simulink model "Model_sim"  (R2018b)
settings: Solver=ode3  StartTime=0.0  StopTime=0.08  FixedStep=0.02  RelTol=1e-3
values from neighbouring files (symbols this model uses):
  q1_d_in = xd0(1,2)    [Project.m]    (also in definitivo.mat = -0.537500213816)
  q1_in = xi0(1,2)    [Project.m]    (also in definitivo.mat = 4.84978546313)
  q2_d_in = xd0(2,2)    [Project.m]    (also in definitivo.mat = 1.25712801049)
  q2_in = xi0(2,2)    [Project.m]    (also in definitivo.mat = 0.122900974203)
  Ts = 1/fs    (= 0.02)    [Project.m]    (also in definitivo.mat)
settings Model: Creator=Andrea Ghezzi  LastModifiedBy=sl65b

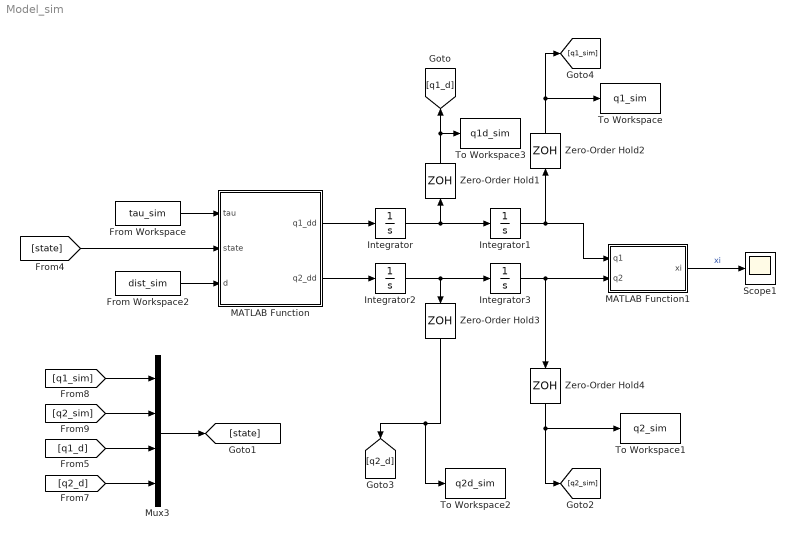
== system Model_sim ==
  From Workspace : FromWorkspace  VariableName=tau_sim  SampleTime=0
  From Workspace2 : FromWorkspace  VariableName=dist_sim  SampleTime=0
  Integrator : Integrator  InitialCondition=q1_d_in
  Integrator1 : Integrator  InitialCondition=q1_in
  Integrator2 : Integrator  InitialCondition=q2_d_in
  Integrator3 : Integrator  InitialCondition=q2_in
  MATLAB Function : MATLAB Function  TreatAsAtomicUnit=on
  MATLAB Function1 : MATLAB Function  TreatAsAtomicUnit=on
  Mux3 : Mux
  Scope1 : Scope
  To Workspace : ToWorkspace  VariableName=q1_sim  SampleTime=-1
  To Workspace1 : ToWorkspace  VariableName=q2_sim  SampleTime=-1
  To Workspace2 : ToWorkspace  VariableName=q2d_sim  SampleTime=-1
  To Workspace3 : ToWorkspace  VariableName=q1d_sim  SampleTime=-1
  Zero-Order Hold{1..4} (4 alike) : ZeroOrderHold  SampleTime=Ts
  wires:
  MATLAB Function/1(q1_dd) -> Integrator/1
  Integrator2/1 -> Integrator3/1, Zero-Order Hold3/1
  Integrator/1 -> Integrator1/1, Zero-Order Hold1/1
  Zero-Order Hold3/1 -> To Workspace2/1, [q2_d]
  Integrator1/1 -> MATLAB Function1/1(q1), Zero-Order Hold2/1
  Integrator3/1 -> MATLAB Function1/2(q2), Zero-Order Hold4/1
  From Workspace/1 -> MATLAB Function/1(tau)
  From Workspace2/1 -> MATLAB Function/3(d)
  MATLAB Function1/1(xi) -> Scope1/1  "xi"
  Zero-Order Hold1/1 -> [q1_d], To Workspace3/1
  Zero-Order Hold4/1 -> [q2_sim], To Workspace1/1
  MATLAB Function/2(q2_dd) -> Integrator2/1
  Zero-Order Hold2/1 -> [q1_sim], To Workspace/1
  Mux3/1 -> [state]
  [state] -> MATLAB Function/2(state)
  [q1_d] -> Mux3/3
  [q2_d] -> Mux3/4
  [q2_sim] -> Mux3/2
  [q1_sim] -> Mux3/1

== matlab function Model_sim/MATLAB Function ==
  data: tau input; state input; d input; q1_dd output; q2_dd output
function [q1_dd, q2_dd] = dynamics(tau, state, d)

F_hx = d(1);
F_hz = d(2);
m_load = d(3);
q1  = state(1);
q2 = state(2);
q1_d = state(3);
q2_d = state(4); 

%robot parameters
g   = 9.81;
J1  = 10;   %inertia link 1
J2  = 10;   %inertia link 2
m1  = 50;   %mass link 1
m2  = 50;   %mass link 2
a1  = 1.2;    %lenght link 1
a2  = 1;  %length link 2
ac1  = a1/2; %centre of mass link 1
ac2  = a2/2; %centre of mass link 2

%kinematic functions
% q1          = q(1);
% q2          = q(2);
% q1_d        = q_d(1);
% q2_d        = q_d(2);
c1          = cos(q1);
s1          = sin(q1);
c2          = cos(q2);
s2          = sin(q2);
c12         = cos(q1+q2);
s12         = sin(q1+q2);

J        = [-a1*sin(q1)-a2*sin(q1+q2)  -a2*sin(q1+q2);
             a1*cos(q1)+a2*cos(q1+q2)   a2*cos(q1+q2)];
         
M_tot =  [m1*ac1^2+m2*(a1^2+ac2^2+2*a1*ac2*c2)+J1+J2     m2*(ac2^2+a1*ac2*c2)+J2;
              m2*(ac2^2+a1*ac2*c2)+J2                    m2*ac2^2+J2];
              
% C_tot = [-a1*q2_d*s2*ac2*m2   -a1*q1_d*s2*ac2*m2;
%           -a1*q1_d*s2*ac2*m2             0];
%- C_tot*[q1_d;q2_d]
         
g_tot = [(m1*ac1+m2*a1)*g*c1+m2*g*ac2*c12;
            m2*g*ac2*c12];
% 

 %equation of motion of the 2dof manipulator 
q_dd = M_tot\(tau + J'*[F_hx;F_hz-m_load*g]- g_tot);
q1_dd = q_dd(1);
q2_dd = q_dd(2);
 
end

== matlab function Model_sim/MATLAB Function1 ==
  data: q1 input; xi output; q2 input
function xi  = direct_kin(q1, q2)
%robot parameters
a1  = 1.2;    %lenght link 1
a2  = 1;  %length link 2

%kinematic functions
c1= cos(q1);
s1= sin(q1);
c2= cos(q2);
s2= sin(q2);
c12= cos(q1+q2);
s12= sin(q1+q2);

% Computation of end effector quantities given the measure joints
% quantities
if q1 == 0 && q2 == 0
    xe = 0;
    ze = 0;
   
else 
    xe = 0.5 + a1*c1 + a2*c12;
    ze = a1*s1 + a2*s12;
    
end
    xi = [xe;ze];
   
end
